simulink model "JenaFox_Hardware"  (R2022a)
settings: Solver=FixedStepAuto  StartTime=0.0  StopTime=inf  FixedStep=hard_step_length  MaxStep=maxStep  RelTol=1e-3  AbsTol=absTol
PreLoadFcn:
  | addpath(genpath("scripts/"));
  | Fox_param;
InitFcn:
  | addpath(genpath("scripts/"));
  | Fox_param;
StartFcn:
  | disp("The robot will now begin to move.")
StopFcn:
  | %Fox_end;
  | disp('Output variables have been saved in XML file.')
undefined symbols (not defined in the file): coms_size_in, coms_size_out, d_cont, f, hard_comsRate, hard_comsRate_controller_in, hard_comsRate_robot_in, hard_comsRate_robot_out, hard_pid_disable, local_ports, mn, National_Instruments, p_cont, PCIe, remote_ports, Standard_Devices, UDP_Protocol
libraries: eeGeneralControl x8, simulink x6, simulink_extras x6, sldrtlib x4, etargetslib x2, instrumentlib x2, slrealtimeiplib x1, slpidlib x1
settings Model: ExtModeTrigDuration=100000  ExtModeLogAll=off  Creator=Fox I (Daniel)  LastModifiedBy=fesch
settings SolverCC: AlgebraicLoopSolver=TrustRegion
settings DataIOCC: ReturnWorkspaceOutputs=off
settings OptimizationCC: EfficientTunableParamExpr=on
settings DebuggingCC: UnconnectedInputMsg=warning  UnconnectedOutputMsg=warning  UnconnectedLineMsg=warning  SFMachineParentedDataDiag=warning  ArithmeticOperatorsInVariantConditions=warning
settings HardwareCC: ProdBitPerLong=64  ProdHWDeviceType=Intel->x86-64 (Linux 64)
settings SFSimCC: SimUseLocalCustomCode=off  CustomCodeUndefinedFunction=UseInterfaceOnly
settings RTWCC: Description=Simulink Desktop Real-Time (ERT)  SystemTargetFile=sldrtert.tlc  TemplateMakefile=sldrtert.tmf  RTWUseLocalCustomCode=off  RTWCompilerOptimization=on
settings CodeAppCC: MaxIdLength=95
settings SimulinkDesktopRealTimeERTCC: TargetFcnLib=ansi_tfl_table_tmw.mat  TargetLibSuffix=_sldrt.a  TargetPreCompLibLocation=C:\Program Files\MATLAB\R2022a\toolbox\sldrt\lib\win64  GenFloatMathFcnCalls=NOT IN USE  TargetLangStandard=C99 (ISO)  CodeReplacementLibrary=None  UtilityFuncGeneration=Auto  MultiwordTypeDef=System defined  MultiwordLength=2048  DynamicStringBufferSize=256  GenerateFullHeader=on  InferredTypesCompatibility=off  GenerateSampleERTMain=off  GenerateTestInterfaces=off  ModelReferenceCompliant=on  ParMdlRefBuildCompliant=off  CompOptLevelCompliant=on  ConcurrentExecutionCompliant=off  IncludeMdlTerminateFcn=on  CombineOutputUpdateFcns=off  CombineSignalStateStructs=off  GroupInternalDataByFunction=off  SuppressErrorStatus=off  IncludeFileDelimiter=Auto  ERTCustomFileBanners=off  SupportAbsoluteTime=on  LogVarNameModifier=rt_  MatFileLogging=off  CodeInterfacePackaging=Nonreusable function  PurelyIntegerCode=off  SupportNonFinite=on  SupportComplex=on  SupportContinuousTime=on  SupportNonInlinedSFcns=on  RemoveDisableFunc=off  RemoveResetFunc=off  SupportVariableSizeSignals=on  ParenthesesLevel=Nominal  CastingMode=Nominal  MATLABClassNameForMDSCustomization=Simulink.SoftwareTarget.TargetSpecificTriggerConfigurationBase  ModelStepFunctionPrototypeControlCompliant=off  CPPClassGenCompliant=off  AutosarCompliant=off  MDXCompliant=off  GRTInterface=off  GenerateAllocFcn=off  UseToolchainInfoCompliant=off  GenerateSharedConstants=on  CoderGroups=[]  AccessMethods=[]  LookupTableObjectStructAxisOrder=1,2,3,4,...  LUTObjectStructOrderExplicitValues=Size,Breakpoints,Table  LUTObjectStructOrderEvenSpacing=Size,Breakpoints,Table  ArrayLayout=Column-major  UnsupportedSFcnMsg=error  ERTHeaderFileRootName=$R$E  ERTSourceFileRootName=$R$E  ERTDataFileRootName=$R_data  OptimizeReductions=off  GenerateASAP2=off  DSAsUniqueAccess=off  InlinedParameterPlacement=Hierarchical  TargetOS=BareBoardExample  MultiInstanceErrorCode=Error  RootIOFormat=Individual arguments  RTWCAPISignals=off  RTWCAPIParams=off  RTWCAPIStates=off  RTWCAPIRootIO=off  ERTSrcFileBannerTemplate=ert_code_template.cgt  ERTHdrFileBannerTemplate=ert_code_template.cgt  ERTDataSrcFileTemplate=ert_code_template.cgt  ERTDataHdrFileTemplate=ert_code_template.cgt  ERTCustomFileTemplate=example_file_process.tlc  EnableDataOwnership=off  SignalDisplayLevel=10  ParamTuneLevel=10  GlobalDataDefinition=Auto  DataDefinitionFile=global.c  GlobalDataReference=Auto  ERTFilePackagingFormat=Modular  RateTransitionBlockCode=Inline  DataReferenceFile=global.h  PreserveExpressionOrder=off  PreserveIfCondition=off  ConvertIfToSwitch=off  PreserveExternInFcnDecls=on  PreserveStaticInFcnDecls=on  SuppressUnreachableDefaultCases=off  EnableSignedLeftShifts=on  EnableSignedRightShifts=on  ImplementImageWithCVMat=off  IndentStyle=K&R  IndentSize=2  NewlineStyle=Default  MaxLineWidth=80  EnableUserReplacementTypes=off  MaxIdInt64=MAX_int64_T  MinIdInt64=MIN_int64_T  MaxIdUint64=MAX_uint64_T  MaxIdInt32=MAX_int32_T  MinIdInt32=MIN_int32_T  MaxIdUint32=MAX_uint32_T  MaxIdInt16=MAX_int16_T  MinIdInt16=MIN_int16_T  MaxIdUint16=MAX_uint16_T  MaxIdInt8=MAX_int8_T  MinIdInt8=MIN_int8_T  MaxIdUint8=MAX_uint8_T  BooleanTrueId=true  BooleanFalseId=false  MemSecPackage=--- None ---  MemSecDataConstants=Default  MemSecDataIO=Default  MemSecDataInternal=Default  MemSecDataParameters=Default  MemSecFuncInitTerm=Default  MemSecFuncExecute=Default  MemSecFuncSharedUtil=Default  GroupConstants=Default  GroupRootInputs=Default  GroupRootOutputs=Default  GroupInternal=Default  GroupParameters=Default  GroupDataTransfer=Default  GroupSharedLocalDataStores=Default  GroupInstanceSpecificParameters=Default  GroupModelData=Default  ArrayContainerType=C-style array  CCListing=off  RebuildAll=off  ExtMode=on  ExtModeTransport=0  ExtModeStaticAlloc=off  ExtModeStaticAllocSize=1000000  ExtModeTesting=off  ExtModeMexFile=sldrtext  ExtModeIntrfLevel=Level1

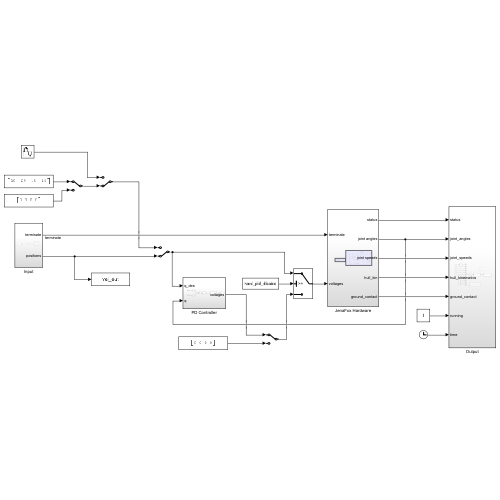
[thumbnail: Simulink's stored preview of the top-level diagram]
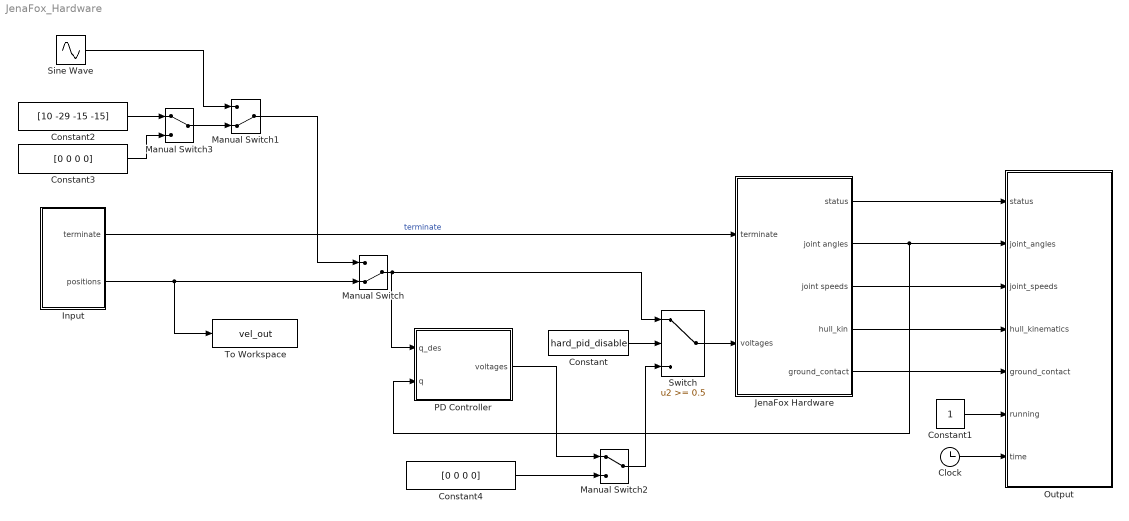
== system JenaFox_Hardware ==
  Clock : Clock
  Constant : Constant  Value=hard_pid_disable
  Constant1 : Constant
  Constant2 : Constant  Value=[10 -29 -15 -15]
  Constant3 : Constant  Value=[0 0 0 0]
  Constant4 : Constant  Value=[0 0 0 0]
  Input : Subsystem
  JenaFox Hardware : Subsystem
  Manual Switch : ManualSwitch  CurrentSetting=0
  Manual Switch1 : ManualSwitch  CurrentSetting=0
  Manual Switch2 : ManualSwitch
  Manual Switch3 : ManualSwitch
  Output : Subsystem
  PD Controller : Subsystem
  Sine Wave : Sin  Amplitude=60  Frequency=pi/1
  Switch : Switch  Threshold=0.5  SaturateOnIntegerOverflow=off  InputSameDT=off
  To Workspace : ToWorkspace  VariableName=vel_out  SaveFormat=Timeseries  SampleTime=-1
  wires:
  Constant/1 -> Switch/2
  Manual Switch/1 -> PD Controller/1(q_des), Switch/1
  PD Controller/1(voltages) -> Manual Switch2/1
  Clock/1 -> Output/7(time)
  Constant1/1 -> Output/6(running)
  JenaFox Hardware/2(joint angles) -> PD Controller/2(q), Output/2(joint_angles)
  Input/1(terminate) -> JenaFox Hardware/1(terminate)  "terminate"
  Switch/1 -> JenaFox Hardware/2(voltages)
  JenaFox Hardware/1(status) -> Output/1(status)
  JenaFox Hardware/3(joint speeds) -> Output/3(joint_speeds)
  JenaFox Hardware/4(hull_kin) -> Output/4(hull_kinematics)
  JenaFox Hardware/5(ground_contact) -> Output/5(ground_contact)
  Manual Switch1/1 -> Manual Switch/1
  Sine Wave/1 -> Manual Switch1/1
  Constant4/1 -> Manual Switch2/2
  Manual Switch2/1 -> Switch/3
  Constant2/1 -> Manual Switch3/1
  Manual Switch3/1 -> Manual Switch1/2
  Constant3/1 -> Manual Switch3/2
  Input/2(positions) -> To Workspace/1, Manual Switch/2

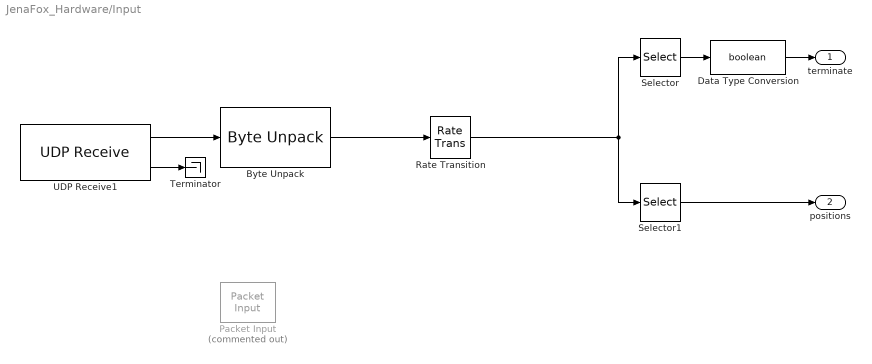
== system JenaFox_Hardware/Input ==
  Byte Unpack : etargetslib/Byte Unpack  dimensions={[coms_size_in/8]}  datatypes={'double'}  byteAlign=1
  Data Type Conversion : DataTypeConversion  OutDataTypeStr=boolean  SaturateOnIntegerOverflow=off  RndMeth=Floor
  Packet Input : sldrtlib/Packet Input  Commented=on  SampleTime=hard_comsRate / 100  MaxMissedTicks=10000  ShowMissedTicks=off  YieldWhenWaiting=off  DrvName=Standard_Devices/UDP_Protocol  DrvAddress=52003  DrvOptions=[0 52002 108 111 99 97 108 104 111 115 116 0 0 0 0 0 0 0 0 0 0 0 0 0 0 0 0 0 0 0 0 0 0 0 0 0 0 0 0 0 0 0 0 0 0 0 0 0 0 0 0 0 0 0 0 0 0 0 0 0 0 0 0 0 0 0 0 0 0 0 0 0 0 0 0 0 0 0 0 0 0 0 0 0 0 0 0 0 0 0 0 0 0 0 0 0 0 0 0 0 0 0 0 0 0 0 0 0 0 0 0 0 0 0 0 0 0 0 0 0 0 0 0 0 0 0 0 0 0 0 0 0 0 0 0 0 0 0 0 0 0 0 0 0 0 0 0 0 0 0 0 0 0 0 0 0 0 0 0 0 0 0 0 0 0 0 0 0 0 0 0 0 0 0 0 0 0 0 0 0 0 0 0 0 0 0 0 0 0 0 0 0 0 0 0 0 0 0 0 0 0 0 0 0 0 0 0 0 0 0 0 0 0 0 0 0 0 0 0 0 0 0 0 0 0 0 0 0 0 0 0 0 0 0 0 0 0 0 0 0 0 0 0 0 0 0 0 0 0 0 0 0 0 0 0 0]  PacketSize=coms_size_in  DataTypes='5*double'  ShowReady=off  ShowError=off  PacketID=1  ByteOrder=1  ShowTimestamp=off
      settings: AttributesFormatString=UDP Protocol [52003]
  Rate Transition : RateTransition  Deterministic=off  OutPortSampleTime=hard_step_length
  Selector : Selector  InputPortWidth=5  IndexOptions=Index vector (dialog)  Indices=[1]  OutputSizes=1
  Selector1 : Selector  InputPortWidth=5  IndexOptions=Index vector (dialog)  Indices=[2 3 4 5]  OutputSizes=1
  Terminator : Terminator
  UDP Receive1 : instrumentlib/UDP Receive  Host=localhost  Port=remote_ports(1)  LocalPort=local_ports(1)  EnablePortSharing=off  GetLatestData=on  DataSize="[coms_size_in   1]"  DataType=uint8  ASCIIFormatting=%f,  Terminator=LF  ByteOrder=BigEndian  EnableBlockingMode=off  Timeout=10  SampleTime=hard_comsRate_controller_in  LocalAddress=0.0.0.0
  terminate : Outport
  positions : Outport  Port=2
  wires:
  UDP Receive1/2 -> Terminator/1
  Byte Unpack/1 -> Rate Transition/1
  Selector1/1 -> positions/1
  Selector/1 -> Data Type Conversion/1
  Data Type Conversion/1 -> terminate/1
  UDP Receive1/1 -> Byte Unpack/1
  Rate Transition/1 -> Selector/1, Selector1/1

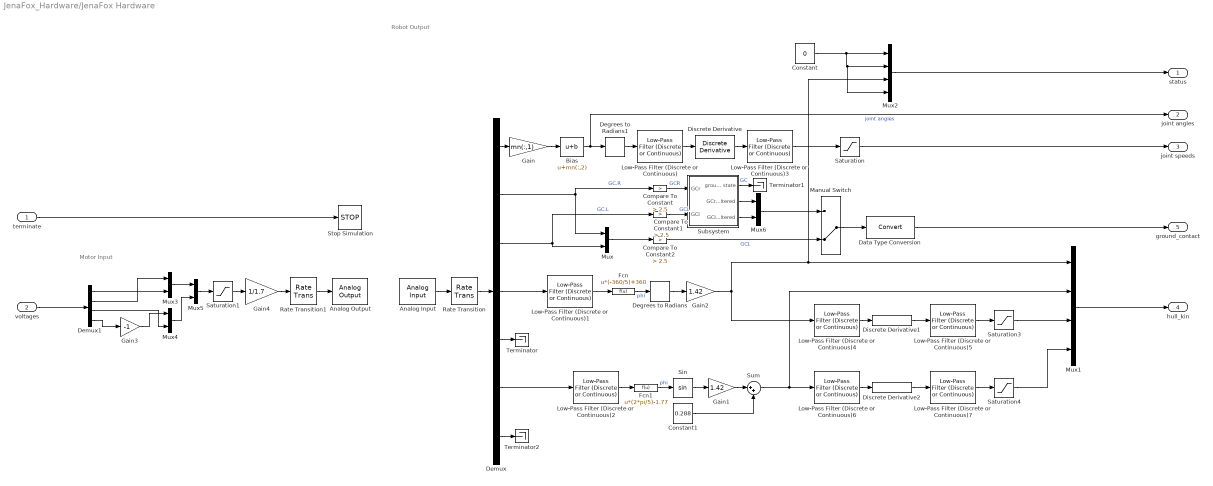
== system JenaFox_Hardware/JenaFox Hardware ==
  note: Motor Input
  note: Robot Output
  terminate : Inport
  voltages : Inport  Port=2
  Analog Input : sldrtlib/Analog Input  SampleTime=hard_comsRate_robot_out  MaxMissedTicks=10000000  ShowMissedTicks=off  YieldWhenWaiting=on  DrvName=National_Instruments/PCIe-6363  DrvAddress=4294967295  DrvOptions=[0 0 0 0 0 0 0]  Channels="[1 2 3 4 5 6 7  29 30 17 18 19 20]"  RangeMode=1  VoltRange=1  DataType=1
      settings: AttributesFormatString=National Instruments\nPCIe-6363 [auto]
  Analog Output : sldrtlib/Analog Output  SampleTime=hard_comsRate_robot_in  MaxMissedTicks=10000000  ShowMissedTicks=off  YieldWhenWaiting=on  DrvName=National_Instruments/PCIe-6363  DrvAddress=4294967295  DrvOptions=[0 0 0 0 0 0 0]  Channels=[1 2 3 4]  RangeMode=1  VoltRange=1  InitialValue=[0 0 0 0]  FinalValue=[0 0 0 0]
      settings: AttributesFormatString=National Instruments\nPCIe-6363 [auto]
  Bias : Bias  Bias=mn(:,2)  SaturateOnIntegerOverflow=off
  Compare To Constant : simulink/Logic and Bit Operations/Compare To Constant  relop=>  const=2.5  OutDataTypeStr=boolean
  Compare To Constant1 : simulink/Logic and Bit Operations/Compare To Constant  relop=>  const=2.5  OutDataTypeStr=boolean
  Compare To Constant2 : simulink/Logic and Bit Operations/Compare To Constant  relop=>  const=2.5  OutDataTypeStr=boolean
  Constant : Constant  Value=0
  Constant1 : Constant  Value=0.288
  Data Type Conversion : DataTypeConversion  SaturateOnIntegerOverflow=off  RndMeth=Floor
  Degrees to Radians : simulink_extras/Transformations/Degrees to Radians
  Degrees to Radians1 : simulink_extras/Transformations/Degrees to Radians
  Demux : Demux  Outputs=[4, 1, 1, 1, 1, 1, 4]
  Demux1 : Demux
  Discrete Derivative : simulink/Discrete/Discrete Derivative  gainval=1  ICPrevScaledInput=0.0  OutMin=[]  OutMax=[]  OutDataType=fixdt(1, 16)  OutScaling=2^-10  DoSatur=off
  Discrete Derivative1 : simulink/Discrete/Discrete Derivative  gainval=1  ICPrevScaledInput=0.0  OutMin=[]  OutMax=[]  OutDataType=fixdt(1, 16)  OutScaling=2^-10  DoSatur=off
  Discrete Derivative2 : simulink/Discrete/Discrete Derivative  gainval=1.0  ICPrevScaledInput=0.0  OutMin=[]  OutMax=[]  OutDataType=fixdt(1, 16)  OutScaling=2^-10  DoSatur=off
  Fcn : Fcn  Expr=u*(-360/5)+360
  Fcn1 : Fcn  Expr=u*(2*pi/5)-1.77
  Gain : Gain  Gain=mn(:,1)
  Gain1 : Gain  Gain=1.42
  Gain2 : Gain  Gain=1.42
  Gain3 : Gain  Gain=-1
  Gain4 : Gain  Gain=1/1.7
  Low-Pass Filter (Discrete or Continuous){,1..7} (8 alike) : eeGeneralControl/Low-Pass Filter (Discrete or Continuous)  K=1  T=1/55  B=inf  A=-inf  init_option=Inherited from block input  x0=0  Ts=-1
  Manual Switch : ManualSwitch  CurrentSetting=0
  Mux{,3..6} (5 alike) : Mux  Inputs=2
  Mux1 : Mux
  Mux2 : Mux
  Rate Transition : RateTransition  Deterministic=off  OutPortSampleTime=hard_step_length
  Rate Transition1 : RateTransition  Deterministic=off  OutPortSampleTime=hard_comsRate_robot_in
  Saturation : Saturate  UpperLimit=44  LowerLimit=-44
  Saturation1 : Saturate  UpperLimit=5.5  LowerLimit=-5.5
  Saturation3 : Saturate  UpperLimit=3  LowerLimit=-3
  Saturation4 : Saturate  UpperLimit=5  LowerLimit=-5
  Sin : Trigonometry
  Stop Simulation : Stop
  Subsystem : Subsystem
  Sum : Sum  Inputs=|++
  Terminator : Terminator
  Terminator1 : Terminator
  Terminator2 : Terminator
  status : Outport
  joint angles : Outport  Port=2
  joint speeds : Outport  Port=3
  hull_kin : Outport  Port=4
  ground_contact : Outport  Port=5
  wires:
  terminate/1 -> Stop Simulation/1
  Mux/1 -> Compare To Constant2/1
  Discrete Derivative/1 -> Low-Pass Filter (Discrete or Continuous)3/1
  Mux2/1 -> status/1
  Mux1/1 -> hull_kin/1
  Manual Switch/1 -> Data Type Conversion/1
  Constant/1 -> Mux2/4, Mux2/2, Mux2/1
  Discrete Derivative2/1 -> Low-Pass Filter (Discrete or Continuous)7/1
  Discrete Derivative1/1 -> Low-Pass Filter (Discrete or Continuous)5/1
  Degrees to Radians/1 -> Gain2/1
  Sum/1 -> Mux1/2, Low-Pass Filter (Discrete or Continuous)6/1
  Sin/1 -> Gain1/1
  Fcn1/1 -> Sin/1  "phi"
  Demux/5 -> Terminator/1
  Fcn/1 -> Degrees to Radians/1  "phi"
  Bias/1 -> Degrees to Radians1/1, joint angles/1  "joint angles"
  Demux/3 -> Compare To Constant1/1, Mux/2  "GC.L"
  Demux/1 -> Gain/1
  Demux/2 -> Compare To Constant/1, Mux/1  "GC.R"
  Demux/4 -> Low-Pass Filter (Discrete or Continuous)1/1
  Compare To Constant/1 -> Subsystem/1("GCr ")  "GCR"
  Analog Input/1 -> Rate Transition/1
  Gain/1 -> Bias/1
  voltages/1 -> Demux1/1
  Mux3/1 -> Mux5/1
  Demux1/3 -> Mux4/2
  Gain3/1 -> Mux4/1
  Demux1/2 -> Mux3/1
  Demux1/1 -> Mux3/2
  Mux5/1 -> Saturation1/1
  Gain4/1 -> Rate Transition1/1
  Demux1/4 -> Gain3/1
  Subsystem/1(ground state) -> Terminator1/1  "GC"
  Subsystem/2(GCr_filtered) -> Mux6/1
  Subsystem/3(GCl_filtered) -> Mux6/2
  Mux6/1 -> Manual Switch/1
  Compare To Constant1/1 -> Subsystem/2("GCl ")  "GCL"
  Rate Transition1/1 -> Analog Output/1
  Compare To Constant2/1 -> Manual Switch/2  "GCL"
  Data Type Conversion/1 -> ground_contact/1
  Gain1/1 -> Sum/1
  Constant1/1 -> Sum/2
  Saturation/1 -> joint speeds/1
  Rate Transition/1 -> Demux/1
  Low-Pass Filter (Discrete or Continuous)1/1 -> Fcn/1
  Saturation3/1 -> Mux1/3
  Demux/6 -> Low-Pass Filter (Discrete or Continuous)2/1
  Saturation4/1 -> Mux1/4
  Mux4/1 -> Mux5/2
  Saturation1/1 -> Gain4/1
  Low-Pass Filter (Discrete or Continuous)/1 -> Discrete Derivative/1
  Low-Pass Filter (Discrete or Continuous)3/1 -> Saturation/1
  Gain2/1 -> Mux2/3, Mux1/1, Low-Pass Filter (Discrete or Continuous)4/1
  Low-Pass Filter (Discrete or Continuous)4/1 -> Discrete Derivative1/1
  Low-Pass Filter (Discrete or Continuous)5/1 -> Saturation3/1
  Low-Pass Filter (Discrete or Continuous)2/1 -> Fcn1/1
  Low-Pass Filter (Discrete or Continuous)6/1 -> Discrete Derivative2/1
  Low-Pass Filter (Discrete or Continuous)7/1 -> Saturation4/1
  Degrees to Radians1/1 -> Low-Pass Filter (Discrete or Continuous)/1
  Demux/7 -> Terminator2/1

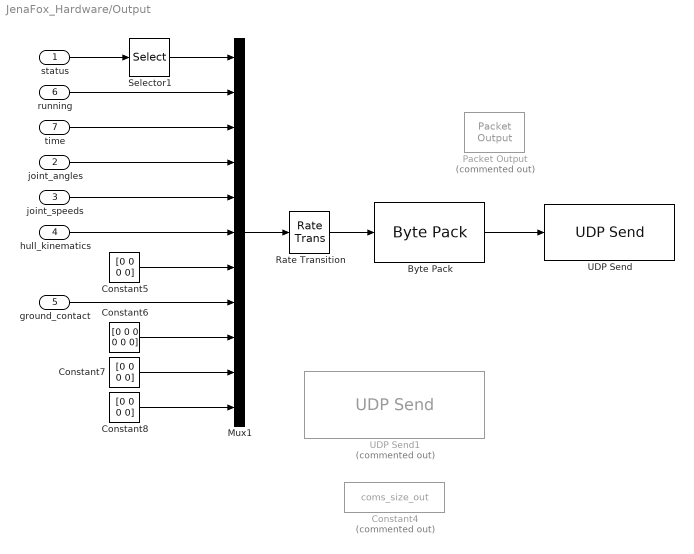
== system JenaFox_Hardware/Output ==
  status : Inport
  joint_angles : Inport  Port=2
  joint_speeds : Inport  Port=3
  hull_kinematics : Inport  Port=4
  ground_contact : Inport  Port=5
  running : Inport  Port=6
  time : Inport  Port=7
  Byte Pack : etargetslib/Byte Pack  datatypes={'double'}  byteAlign=1
  Constant4 : Constant  Commented=on  Value=coms_size_out
  Constant5 : Constant  Value=[0 0 0 0]
  Constant6 : Constant  Value=[0 0 0 0 0 0]
  Constant7 : Constant  Value=[0 0 0 0]
  Constant8 : Constant  Value=[0 0 0 0]
  Mux1 : Mux  Inputs=11
  Packet Output : sldrtlib/Packet Output  Commented=on  SampleTime=hard_comsRate  MaxMissedTicks=10000  ShowMissedTicks=off  YieldWhenWaiting=on  DrvName=Standard_Devices/UDP_Protocol  DrvAddress=52000  DrvOptions=[0 52001 108 111 99 97 108 104 111 115 116 0 0 0 0 0 0 0 0 0 0 0 0 0 0 0 0 0 0 0 0 0 0 0 0 0 0 0 0 0 0 0 0 0 0 0 0 0 0 0 0 0 0 0 0 0 0 0 0 0 0 0 0 0 0 0 0 0 0 0 0 0 0 0 0 0 0 0 0 0 0 0 0 0 0 0 0 0 0 0 0 0 0 0 0 0 0 0 0 0 0 0 0 0 0 0 0 0 0 0 0 0 0 0 0 0 0 0 0 0 0 0 0 0 0 0 0 0 0 0 0 0 0 0 0 0 0 0 0 0 0 0 0 0 0 0 0 0 0 0 0 0 0 0 0 0 0 0 0 0 0 0 0 0 0 0 0 0 0 0 0 0 0 0 0 0 0 0 0 0 0 0 0 0 0 0 0 0 0 0 0 0 0 0 0 0 0 0 0 0 0 0 0 0 0 0 0 0 0 0 0 0 0 0 0 0 0 0 0 0 0 0 0 0 0 0 0 0 0 0 0 0 0 0 0 0 0 0 0 0 0 0 0 0 0 0 0 0 0 0 0 0 0 0 0 0]  PacketSize=coms_size_out  DataTypes='15*double'  ShowReady=off  ShowError=off  PacketID=1  ByteOrder=1  InitialValue=[]  FinalValue=[]
      settings: AttributesFormatString=UDP Protocol [52000]
  Rate Transition : RateTransition  Deterministic=off  OutPortSampleTime=hard_comsRate_controller_out
  Selector1 : Selector  InputPortWidth=4  IndexOptions=Index vector (dialog)  Indices=[1 2 3]  OutputSizes=1
  UDP Send : instrumentlib/UDP Send  Host=localhost  Port=remote_ports(2)  LocalPort=local_ports(2)  EnablePortSharing=off  ByteOrder=BigEndian  OutputDatagramPacketSize=coms_size_out  EnableBlockingMode=off  LocalAddress=0.0.0.0
  UDP Send1 : slrealtimeiplib/UDP Send  Commented=on  useHostTargetConn=off  toAddress=255.255.255.255  toPort=remote_ports(2)  sampleTime=-1  enableMessage=off
      settings: SourceProductBaseCode=XP
  wires:
  Constant7/1 -> Mux1/10
  Selector1/1 -> Mux1/1
  Constant5/1 -> Mux1/7
  joint_angles/1 -> Mux1/4
  joint_speeds/1 -> Mux1/5
  ground_contact/1 -> Mux1/8
  running/1 -> Mux1/2
  status/1 -> Selector1/1
  Constant6/1 -> Mux1/9
  Constant8/1 -> Mux1/11
  hull_kinematics/1 -> Mux1/6
  time/1 -> Mux1/3
  Rate Transition/1 -> Byte Pack/1
  Byte Pack/1 -> UDP Send/1
  Mux1/1 -> Rate Transition/1

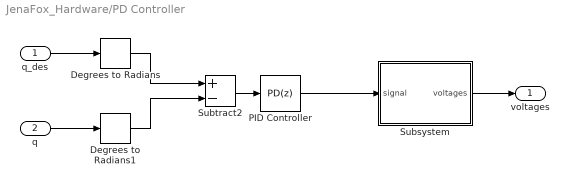
== system JenaFox_Hardware/PD Controller ==
  q_des : Inport
  q : Inport  Port=2
  Degrees to Radians : simulink_extras/Transformations/Degrees to Radians
  Degrees to Radians1 : simulink_extras/Transformations/Degrees to Radians
  PID Controller : slpidlib/PID Controller  Controller=PD  Form=Parallel  TimeDomain=Discrete-time  UseExternalTs=off  SampleTime=-1  IntegratorMethod=Forward Euler  FilterMethod=Forward Euler  ControllerParametersSource=internal  P=p_cont  I=0  UseKiTs=off  D=-d_cont  N=1  UseFilter=on  TunerSelectOption=Transfer Function Based (PID Tuner App)  InitialConditionSource=internal  InitialConditionForIntegrator=0  InitialConditionForFilter=0  DifferentiatorICPrevScaledInput=0  ExternalReset=none  TrackingMode=off  Kt=1  LimitOutput=off  SatLimitsSource=internal  UpperSaturationLimit=inf  LowerSaturationLimit=-inf  LinearizeAsGain=on  AntiWindupMode=none  Kb=1  POutMin=[]  POutMax=[]  IOutMin=[]  IOutMax=[]  DOutMin=[]  DOutMax=[]  NOutMin=[]  NOutMax=[]  SumOutMin=[]  SumOutMax=[]  SaturationOutMin=[]  SaturationOutMax=[]  PParamMin=[]  PParamMax=[]  IParamMin=[]  IParamMax=[]  DParamMin=[]  DParamMax=[]  NParamMin=[]  NParamMax=[]  KbParamMin=[]  KbParamMax=[]  KtParamMin=[]  KtParamMax=[]  KbOutMin=[]  KbOutMax=[]  KtOutMin=[]  KtOutMax=[]  IntegratorOutMin=[]  IntegratorOutMax=[]  FilterOutMin=[]  FilterOutMax=[]  SumI1OutMin=[]  SumI1OutMax=[]  SumI2OutMin=[]  SumI2OutMax=[]  SumI3OutMin=[]  SumI3OutMax=[]  SumI4OutMin=[]  SumI4OutMax=[]  SumDOutMin=[]  SumDOutMax=[]  DifferentiatorOutMin=[]  DifferentiatorOutMax=[]  FilterDiffOutCoefMin=[]  FilterDiffOutCoefMax=[]  ReciprocalOutMin=[]  ReciprocalOutMax=[]  SumDenOutMin=[]  SumDenOutMax=[]  SumNumOutMin=[]  SumNumOutMax=[]  DivideOutMin=[]  DivideOutMax=[]  UdiffTsProdOutMin=[]  UdiffTsProdOutMax=[]  NTsProdOutMin=[]  NTsProdOutMax=[]  UintegralTsProdOutMin=[]  UintegralTsProdOutMax=[]  UngainTsProdOutMin=[]  UngainTsProdOutMax=[]  IntegratorContinuousStateAttributes=''  IntegratorStateMustResolveToSignalObject=off  IntegratorRTWStateStorageClass=Auto  FilterContinuousStateAttributes=''  FilterStateMustResolveToSignalObject=off  FilterRTWStateStorageClass=Auto  ParallelPVariant=InternalParameters  IdealPVariant=Disabled  IVariant=Disabled  DVariant=InternalParameters  IntegratorVariant=Disabled  SatVariant=Disabled  AWVariant=Disabled  PCopyVariant=Disabled  TRVariant=Disabled  FdbkBlocksVariant=Forward  IdealPFdbkVariant=Disabled  SatFdbkVariant=Disabled  DerivativeFilterVariant=ForwardEulerFilter  NVariant=InternalParameters  NCopyVariant=Disabled  FilterICVariant=InternalICsFilter  IntegratorICVariant=Disabled  ExternalResetVariant=Disabled  TRSumVariant=Passthrough  SumFdbkVariant=Disabled  SumVariant=Sum_PD  TsampFilterVariant=InternalTs  TsampNgainVariant=Passthrough  TsampIntegralVariant=Disabled_SignalSpec  ExternalSaturationOutDataTypeStr=Inherit: Same as second input  aMode=0
  Subsystem : Subsystem
  Subtract2 : Sum  Inputs=+-
  voltages : Outport
  wires:
  PID Controller/1 -> Subsystem/1(signal)
  Subtract2/1 -> PID Controller/1
  Degrees to Radians/1 -> Subtract2/1
  q/1 -> Degrees to Radians1/1
  Degrees to Radians1/1 -> Subtract2/2
  q_des/1 -> Degrees to Radians/1
  Subsystem/1(voltages) -> voltages/1

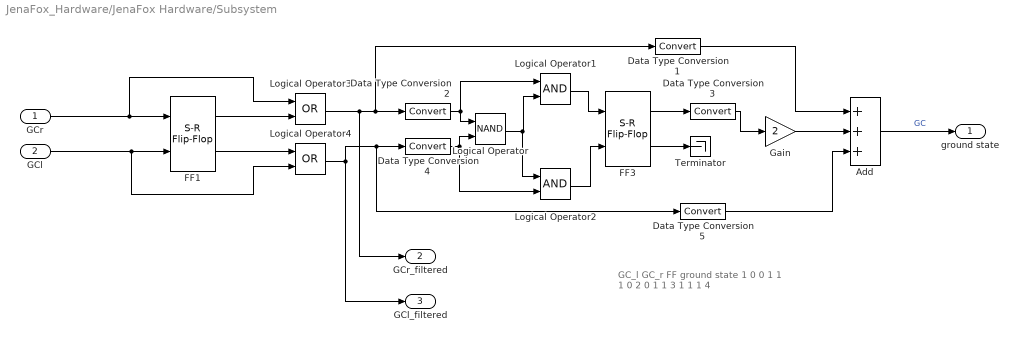
== system JenaFox_Hardware/JenaFox Hardware/Subsystem ==
  note: GC_l   GC_r   FF   ground state
      | 1         0         0       1
      | 1         1         0       2
      | 0         1         1       3
      | 1         1         1       4
  "GCr " : Inport
  "GCl " : Inport  Port=2
  Add : Sum  Inputs=+++
  Data Type Conversion{1..5} (5 alike) : DataTypeConversion  SaturateOnIntegerOverflow=off  RndMeth=Floor
  FF1 : simulink_extras/Flip Flops/S-R Flip-Flop  initial_condition=0
  FF3 : simulink_extras/Flip Flops/S-R Flip-Flop  initial_condition=0
  Gain : Gain  Gain=2
  Logical Operator : Logic  Operator=NAND  AllPortsSameDT=off  OutDataTypeStr=boolean
  Logical Operator1 : Logic  AllPortsSameDT=off  OutDataTypeStr=boolean
  Logical Operator2 : Logic  AllPortsSameDT=off  OutDataTypeStr=boolean
  Logical Operator3 : Logic  Operator=OR  AllPortsSameDT=off  OutDataTypeStr=boolean
  Logical Operator4 : Logic  Operator=OR  AllPortsSameDT=off  OutDataTypeStr=boolean
  Terminator : Terminator
  ground state : Outport  VectorParamsAs1DForOutWhenUnconnected=off
  GCr_filtered : Outport  Port=2
  GCl_filtered : Outport  Port=3
  wires:
  Data Type Conversion1/1 -> Add/1
  Logical Operator4/1 -> GCl_filtered/1, Data Type Conversion5/1, Data Type Conversion4/1
  Logical Operator2/1 -> FF3/2
  Data Type Conversion5/1 -> Add/3
  Logical Operator/1 -> Logical Operator2/1, Logical Operator1/2
  FF3/1 -> Data Type Conversion3/1
  Gain/1 -> Add/2
  Logical Operator3/1 -> GCr_filtered/1, Data Type Conversion1/1, Data Type Conversion2/1
  FF1/2 -> Logical Operator4/1
  Data Type Conversion4/1 -> Logical Operator2/2, Logical Operator/2
  FF1/1 -> Logical Operator3/2
  Data Type Conversion3/1 -> Gain/1
  Data Type Conversion2/1 -> Logical Operator1/1, Logical Operator/1
  FF3/2 -> Terminator/1
  Logical Operator1/1 -> FF3/1
  Add/1 -> ground state/1  "GC"
  "GCl "/1 -> Logical Operator4/2, FF1/2
  "GCr "/1 -> Logical Operator3/1, FF1/1

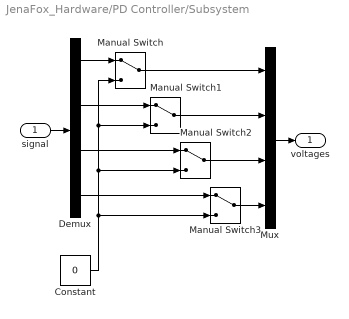
== system JenaFox_Hardware/PD Controller/Subsystem ==
  signal : Inport
  Constant : Constant  Value=0
  Demux : Demux
  Manual Switch{,1..3} (4 alike) : ManualSwitch
  Mux : Mux
  voltages : Outport
  wires:
  Manual Switch/1 -> Mux/1
  Constant/1 -> Manual Switch3/2, Manual Switch2/2, Manual Switch1/2, Manual Switch/2
  Manual Switch2/1 -> Mux/3
  Demux/4 -> Manual Switch3/1
  Manual Switch1/1 -> Mux/2
  Mux/1 -> voltages/1
  Manual Switch3/1 -> Mux/4
  signal/1 -> Demux/1
  Demux/3 -> Manual Switch2/1
  Demux/2 -> Manual Switch1/1
  Demux/1 -> Manual Switch/1
